simulink model "PO"  (Simulink 7.5)
settings: Solver=ode23t  StartTime=0.0  StopTime=1.4  RelTol=1e-3
libraries: powerlib x23, powerlib_extras x6, simulink x3
settings Model: Creator=Raju  LastModifiedBy=Lenovo
settings SolverCC: ZeroCrossControl=DisableAll

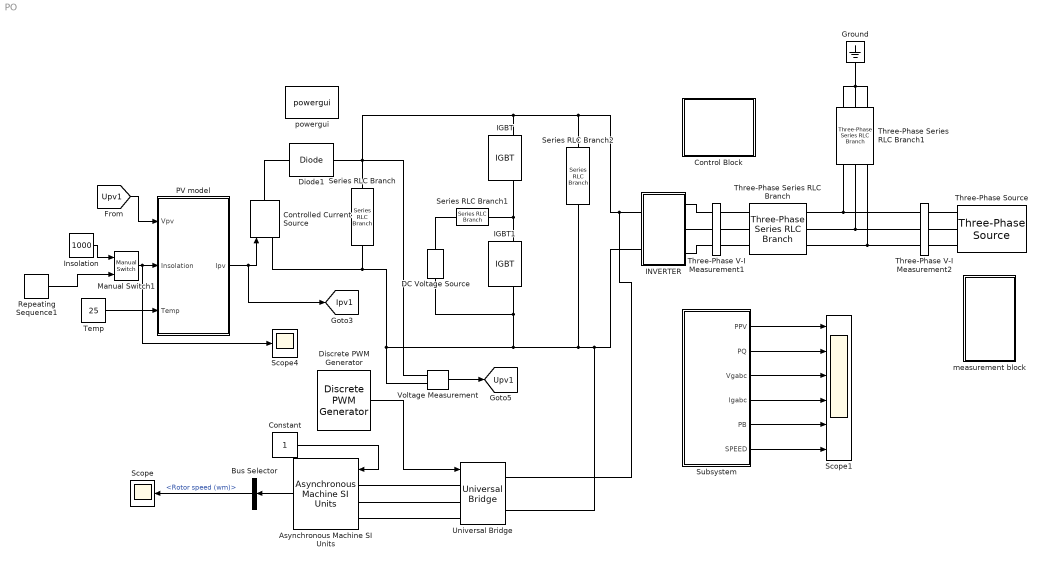
== system PO ==
  " INVERTER" : Subsystem
  Asynchronous Machine SI Units : powerlib/Machines/Asynchronous Machine SI Units  DialogController=POWERSYS.PowerSysDialog  SystemSampleTime=-1  PresetModel=No  MechanicalLoad=Torque Tm  ShowDetailedParameters=on  RotorType=Squirrel-cage  ReferenceFrame=Rotor  NominalParameters=[ 2250*746, 400, 50 ]  Stator=[ 0.029 0.226/377]  Rotor=[ 0.022 0.226/377]  Lm=13.04/377  Mechanical=[ 63.87 0 2]  PolePairs=2  InitialConditions=[1 0 0 0 0 0 0 0]  Units=SI  LoadFlowParameters=1492000  SimulateSaturation=off  Saturation=[14.03593122, 27.81365428, 53.79336849, 72.68890987, 97.98006896, 148.6815601, 215.7428561, 302.9841135, 428.7778367 ; 230, 322, 414, 460, 506, 552, 598, 644, 690]  TsPowergui=0  TsBlock=-1  IterativeModel=Forward Euler
  Bus Selector : BusSelector  OutputSignals=Mechanical.Rotor speed (wm)
  Constant : Constant  OutDataType=fixdt(1, 16)  OutScaling=2^0
  Control Block : Subsystem
  Controlled Current Source : powerlib/Electrical Sources/Controlled Current Source  DialogController=POWERSYS.PowerSysDialog  SystemSampleTime=-1  Initialize=on  Source_Type=AC  Amplitude=0  Phase=0  Frequency=0  Measurements=Current
  DC Voltage Source : powerlib/Electrical Sources/DC Voltage Source  DialogController=POWERSYS.PowerSysDialog  SystemSampleTime=-1  Amplitude=240  Measurements=None
  Diode1 : powerlib/Power Electronics/Diode  DialogController=POWERSYS.PowerSysDialog  SystemSampleTime=-1  Ron=0.001  Lon=0  Vf=0.8  IC=0  UseSnubber=off  Rs=500  Cs=250e-9  Measurements=off
  Discrete PWM Generator : powerlib_extras/Discrete  Control Blocks/Discrete PWM Generator  DialogController=POWERSYS.PowerSysDialog  SystemSampleTime=-1  GeneratorMode="3-arm  bridge (6 pulses)"  Fc=1080  Ts=50e-6  Internal=on  mIndex=0.4  Freq=60  Phase=0
  Ground : powerlib/Elements/Ground  DialogController=POWERSYS.PowerSysDialog  PhysicalDomain=powersysdomain  SubClassName=unknown  LeftPortType=p1  RightPortType=p1  LConnTagsString=a
  IGBT : powerlib/Power Electronics/IGBT  DialogController=POWERSYS.PowerSysDialog  SystemSampleTime=-1  Ron=0.001  Lon=0  Vf=1  Tf=1e-6  Tt=2e-6  IC=0  Rs=1e5  Cs=inf  Measurements=on
  IGBT1 : powerlib/Power Electronics/IGBT  DialogController=POWERSYS.PowerSysDialog  SystemSampleTime=-1  Ron=0.001  Lon=0  Vf=1  Tf=1e-6  Tt=2e-6  IC=0  Rs=1e5  Cs=inf  Measurements=on
  Insolation : Constant  Value=1000
  Manual Switch1 : simulink/Signal Routing/Manual Switch  SystemSampleTime=-1  sw=1  action=0  varsize=off
  PV model : Subsystem
  Repeating Sequence1 : simulink/Sources/Repeating Sequence  SystemSampleTime=-1  rep_seq_t=[0 0.5 0.5 0.8 0.8 1.5 ]  rep_seq_y=[1000 1000 700 700 1000 1000]
  Scope : Scope
  Scope1 : Scope  NumInputPorts=6
      settings: YMin=-5~-5~-5~-5~-5~-5  YMax=5~5~5~5~5~5  SaveName=ScopeData2
  Scope4 : Scope
      settings: YMin=-100  YMax=800  SaveName=v1
  Series RLC Branch : powerlib/Elements/Series RLC Branch  DialogController=POWERSYS.PowerSysDialog  PhysicalDomain=powersysdomain  SubClassName=unknown  LeftPortType=p1  RightPortType=p1  LConnTagsString=__new0  RConnTagsString=__new0  BranchType=C  Resistance=1  Inductance=1e-3  SetiL0=off  InitialCurrent=0  Capacitance=138e-6  Setx0=off  InitialVoltage=0  Measurements=None
  Series RLC Branch1 : powerlib/Elements/Series RLC Branch  DialogController=POWERSYS.PowerSysDialog  PhysicalDomain=powersysdomain  SubClassName=unknown  LeftPortType=p1  RightPortType=p1  LConnTagsString=__new0  RConnTagsString=__new0  BranchType=L  Resistance=1  Inductance=2.2e-3  SetiL0=off  InitialCurrent=0  Capacitance=4700e-6  Setx0=off  InitialVoltage=0  Measurements=None
  Series RLC Branch2 : powerlib/Elements/Series RLC Branch  DialogController=POWERSYS.PowerSysDialog  PhysicalDomain=powersysdomain  SubClassName=unknown  LeftPortType=p1  RightPortType=p1  LConnTagsString=__new0  RConnTagsString=__new0  BranchType=C  Resistance=1  Inductance=1e-3  SetiL0=off  InitialCurrent=0  Capacitance=4700e-6  Setx0=off  InitialVoltage=0  Measurements=None
  Subsystem : Subsystem
  Temp : Constant  Value=25
  Three-Phase Series RLC Branch : powerlib/Elements/Three-Phase Series RLC Branch  DialogController=POWERSYS.PowerSysDialog  PhysicalDomain=powersysdomain  SubClassName=unknown  LeftPortType=p1  RightPortType=p1  LConnTagsString=A|B|C  RConnTagsString=A|B|C  BranchType=L  Resistance=0.5  Inductance=6e-3  Capacitance=1e-6  Measurements=None
  Three-Phase Series RLC Branch1 : powerlib/Elements/Three-Phase Series RLC Branch  DialogController=POWERSYS.PowerSysDialog  PhysicalDomain=powersysdomain  SubClassName=unknown  LeftPortType=p1  RightPortType=p1  LConnTagsString=A|B|C  RConnTagsString=A|B|C  BranchType=RC  Resistance=1  Inductance=1e-3  Capacitance=1e-6  Measurements=None
  Three-Phase V-I Measurement1 : powerlib/Measurements/Three-Phase V-I Measurement  DialogController=POWERSYS.PowerSysDialog  SystemSampleTime=-1  VoltageMeasurement=phase-to-ground  SetLabelV=on  LabelV=Viabc  Vpu=off  VpuLL=off  CurrentMeasurement=yes  SetLabelI=on  LabelI=Iiabc  Ipu=off  Pbase=100e6  Vbase=500e3  OutputType=Complex  PhasorSimulation=off  PSBequivalent=0
      link override Model/VI/Ia: GotoTag=LibraryTag_Ia
      link override Model/VI/Ib: GotoTag=LibraryTag_Ib
      link override Model/VI/Ic: GotoTag=LibraryTag_Ic
      link override Model/VI/Va: GotoTag=LibraryTag_Va
      link override Model/VI/Vb: GotoTag=LibraryTag_Vb
      link override Model/VI/Vc: GotoTag=LibraryTag_Vc
  Three-Phase V-I Measurement2 : powerlib/Measurements/Three-Phase V-I Measurement  DialogController=POWERSYS.PowerSysDialog  SystemSampleTime=-1  VoltageMeasurement=phase-to-phase  SetLabelV=on  LabelV=Vsabc  Vpu=off  VpuLL=off  CurrentMeasurement=yes  SetLabelI=on  LabelI=Isabc  Ipu=off  Pbase=100e6  Vbase=500e3  OutputType=Complex  PhasorSimulation=off  PSBequivalent=0
      link override Model/VI/Ia: GotoTag=LibraryTag_Ia
      link override Model/VI/Ib: GotoTag=LibraryTag_Ib
      link override Model/VI/Ic: GotoTag=LibraryTag_Ic
      link override Model/VI/Va: GotoTag=LibraryTag_Va
      link override Model/VI/Vb: GotoTag=LibraryTag_Vb
      link override Model/VI/Vc: GotoTag=LibraryTag_Vc
  Three-Phase Source : powerlib/Electrical Sources/Three-Phase Source  DialogController=POWERSYS.PowerSysDialog  SystemSampleTime=-1  Voltage=400  PhaseAngle=0  Frequency=50  InternalConnection=Yg  SpecifyImpedance=off  Resistance=0.01  Inductance=2e-6  ShortCircuitLevel=10e6  BaseVoltage=400  XRratio=7
  Universal Bridge : powerlib/Power Electronics/Universal Bridge  DialogController=POWERSYS.PowerSysDialog  SystemSampleTime=-1  Arms=3  SnubberResistance=1e5  SnubberCapacitance=inf  Device=IGBT / Diodes  Ron=1e-3  Lon=0  ForwardVoltages="[  0  0  ]"  ForwardVoltage=0  GTOparameters=[ 10e-6 , 20e-6 ]  IGBTparameters=[ 1e-6 , 2e-6 ]  Measurements=None  Measurements_2=None  converterType=Rectifier
  Voltage Measurement : powerlib/Measurements/Voltage Measurement  DialogController=POWERSYS.PowerSysDialog  SystemSampleTime=-1  PhasorSimulation=off  OutputType=Complex  PSBequivalent=0
  measurement block : Subsystem
  powergui : powerlib/powergui  Priority=1  SystemSampleTime=-1  SimulationMode=Discrete  SampleTime=50e-6  frequency=60  SPID=off  DisableSnubberDevices=off  DisableRonSwitches=off  DisableVfSwitches=off  SwTol=0  Interpol=off  frequencyindice=50  echomessages=off  HookPort=off  DisplayEquations=off  FunctionMessages=off  EnableUseOfTLC=off  x0status=blocks  RestoreLinks=warning  ResistiveCurrentMeasurement=off  Ylog=off  Xlog=on  ShowGrid=off  save=off  variable=ZData  structure=Is  ZoomFFT=off  StartTime=0.5  cycles=1  DisplayStyle=1  fundamental=50  FreqAxis=on  MaxFrequency=5000  frequencyindicesteady=1  display=off  methode=off
  tag scope: Ipv1=global, Upv1=global
  wires:
  PV model/1(Ipv) -> Controlled Current Source/1, [Ipv1]
  Voltage Measurement/1 -> [Upv1]
  Temp/1 -> PV model/3(Temp)
  Manual Switch1/1 -> PV model/2(Insolation), Scope4/1
  Insolation/1 -> Manual Switch1/1
  Repeating Sequence1/1 -> Manual Switch1/2
  [Upv1] -> PV model/1(Vpv)
  Discrete PWM Generator/1 -> Universal Bridge/1
  Asynchronous Machine SI Units/1 -> Bus Selector/1
  Bus Selector/1 -> Scope/1  "<Rotor speed (wm)>"
  Constant/1 -> Asynchronous Machine SI Units/1
  Subsystem/1(PPV) -> Scope1/1
  Subsystem/2(PQ) -> Scope1/2
  Subsystem/3(Vgabc) -> Scope1/3
  Subsystem/4(Igabc) -> Scope1/4
  Subsystem/5(PB) -> Scope1/5
  Subsystem/6(SPEED) -> Scope1/6
  connections:
  Series RLC Branch2/RConn1 -- IGBT1/RConn1 -- DC Voltage Source/LConn1 -- Voltage Measurement/LConn2 -- Controlled Current Source/LConn1 -- Series RLC Branch/RConn1 -- " INVERTER"/LConn2 -- Universal Bridge/RConn2
  " INVERTER"/RConn1 -- Three-Phase V-I Measurement1/LConn1
  " INVERTER"/RConn2 -- Three-Phase V-I Measurement1/LConn2
  " INVERTER"/RConn3 -- Three-Phase V-I Measurement1/LConn3
  Three-Phase V-I Measurement1/RConn1 -- Three-Phase Series RLC Branch/LConn1
  Three-Phase V-I Measurement1/RConn2 -- Three-Phase Series RLC Branch/LConn2
  Three-Phase V-I Measurement1/RConn3 -- Three-Phase Series RLC Branch/LConn3
  Three-Phase Source/RConn1 -- Three-Phase V-I Measurement2/RConn1
  Three-Phase Source/RConn2 -- Three-Phase V-I Measurement2/RConn2
  Three-Phase Source/RConn3 -- Three-Phase V-I Measurement2/RConn3
  Three-Phase Series RLC Branch1/LConn3 -- Three-Phase Series RLC Branch/RConn3 -- Three-Phase V-I Measurement2/LConn3
  Three-Phase Series RLC Branch1/LConn2 -- Three-Phase Series RLC Branch/RConn2 -- Three-Phase V-I Measurement2/LConn2
  Three-Phase Series RLC Branch1/LConn1 -- Three-Phase Series RLC Branch/RConn1 -- Three-Phase V-I Measurement2/LConn1
  Universal Bridge/RConn1 -- Diode1/RConn1 -- Voltage Measurement/LConn1 -- Series RLC Branch/LConn1 -- IGBT/LConn1 -- Series RLC Branch2/LConn1 -- " INVERTER"/LConn1
  Diode1/LConn1 -- Controlled Current Source/RConn1
  IGBT/RConn1 -- IGBT1/LConn1 -- Series RLC Branch1/LConn1
  DC Voltage Source/RConn1 -- Series RLC Branch1/RConn1
  Universal Bridge/LConn1 -- Asynchronous Machine SI Units/LConn1
  Universal Bridge/LConn2 -- Asynchronous Machine SI Units/LConn2
  Universal Bridge/LConn3 -- Asynchronous Machine SI Units/LConn3
  Ground/LConn1 -- Three-Phase Series RLC Branch1/RConn1 -- Three-Phase Series RLC Branch1/RConn3 -- Three-Phase Series RLC Branch1/RConn2

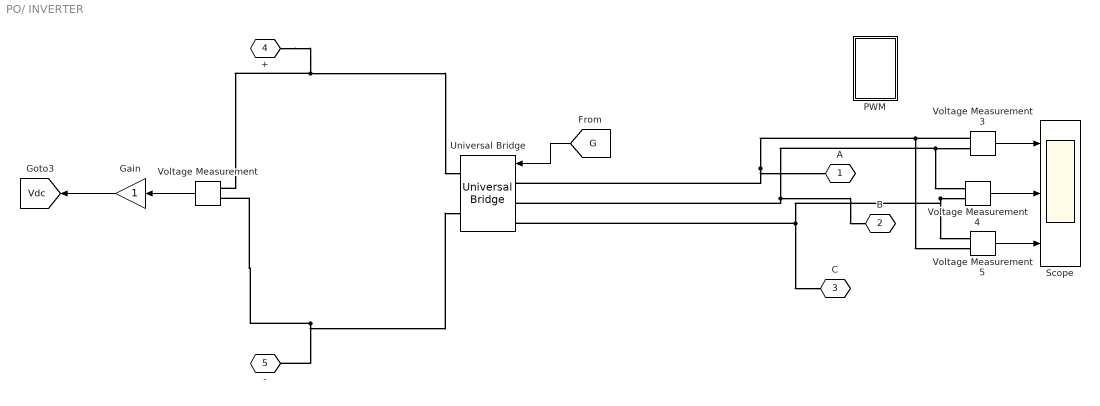
== system PO/ INVERTER ==
  Gain : Gain
  PWM : Subsystem
  Scope : Scope  NumInputPorts=3
      settings: TimeRange=0.1485544839330016  YMin=-300~-400~-300  YMax=300~300~300  SaveName=ScopeData3
  Universal Bridge : powerlib/Power Electronics/Universal Bridge  DialogController=POWERSYS.PowerSysDialog  SystemSampleTime=-1  Arms=3  SnubberResistance=1e5  SnubberCapacitance=inf  Device=IGBT / Diodes  Ron=1e-3  Lon=0  ForwardVoltages="[  0  0  ]"  ForwardVoltage=0  GTOparameters=[ 10e-6 , 20e-6 ]  IGBTparameters=[ 1e-6 , 2e-6 ]  Measurements=None  Measurements_2=None  converterType=Rectifier
  Voltage Measurement{,3..5} (4 alike) : powerlib/Measurements/Voltage Measurement  DialogController=POWERSYS.PowerSysDialog  SystemSampleTime=-1  PhasorSimulation=off  OutputType=Complex  PSBequivalent=0
  A : PMIOPort  Tag=PMCPort  Port=1  Side=Right
  B : PMIOPort  Tag=PMCPort  Port=2  Side=Right
  C : PMIOPort  Tag=PMCPort  Port=3  Side=Right
  + : PMIOPort  Tag=PMCPort  Port=4  Side=Left
  - : PMIOPort  Tag=PMCPort  Port=5  Side=Left
  tag scope: Vdc=global
  wires:
  Voltage Measurement3/1 -> Scope/1
  Voltage Measurement4/1 -> Scope/2
  Voltage Measurement5/1 -> Scope/3
  Voltage Measurement/1 -> Gain/1
  Gain/1 -> [Vdc]
  [G] -> Universal Bridge/1
  connections:
  +/RConn1 -- Voltage Measurement/LConn1 -- Universal Bridge/RConn1
  -/RConn1 -- Voltage Measurement/LConn2 -- Universal Bridge/RConn2
  Voltage Measurement4/LConn2 -- Voltage Measurement5/LConn1 -- C/RConn1 -- Universal Bridge/LConn3
  Voltage Measurement3/LConn2 -- Voltage Measurement4/LConn1 -- B/RConn1 -- Universal Bridge/LConn2
  Voltage Measurement3/LConn1 -- Voltage Measurement5/LConn2 -- A/RConn1 -- Universal Bridge/LConn1

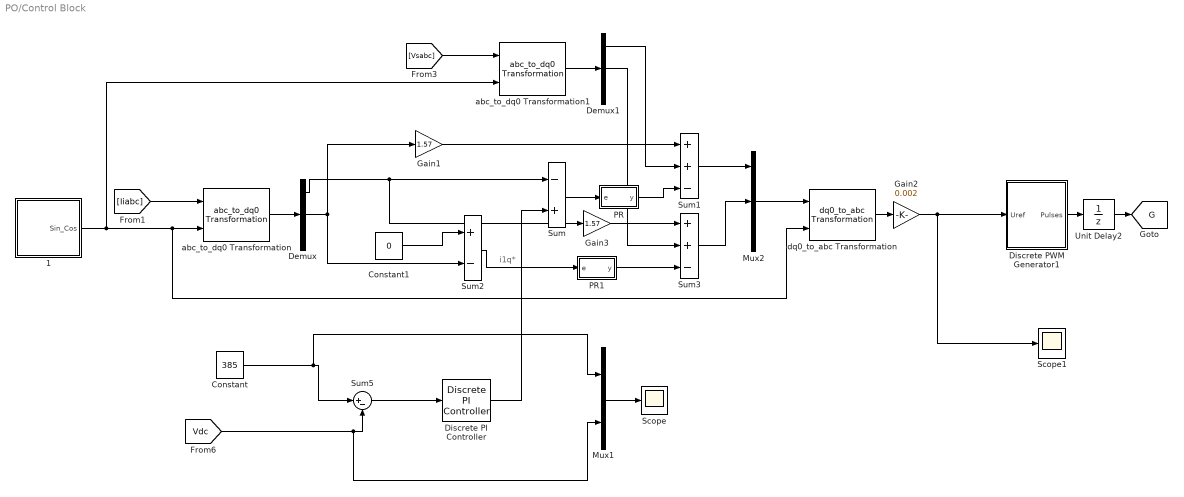
== system PO/Control Block ==
  note: i1q*
  1 : Subsystem
  Constant : Constant  Value=385  OutDataType=fixdt(1, 16)  OutScaling=2^0
  Constant1 : Constant  Value=0  OutDataType=fixdt(1, 16)  OutScaling=2^0
  Demux : Demux  Outputs=3
  Demux1 : Demux  Outputs=3
  Discrete PI Controller : powerlib_extras/Discrete  Control Blocks/Discrete PI Controller  DialogController=POWERSYS.PowerSysDialog  SystemSampleTime=-1  Kp=0.1  Ki=1  Par_Limits=[1e6 -1e6]  Init=0  Ts=50e-6
  Discrete PWM Generator1 : Subsystem  AncestorBlock=|  DialogController=POWERSYS.PowerSysDialog  mask(Discrete PWM Generator){GeneratorMode=3-arm  bridge (6 pulses), Fc=7000, Ts=50e-6, Internal=off, mIndex=0.4, Freq=60, Phase=0}
      | powerlib_extras/Discrete 
      | Control Blocks/Discrete
      | PWM Generator
      mask prompts: GeneratorMode "Generator Mode"; Fc "Carrier frequency (Hz):"; Ts "Sample time:"; Internal "Internal generation of modulating signal(s)"; mIndex "Modulation index  (0<m<1) :"; Freq "Frequency of output voltage (Hz)"; Phase "Phase of output voltage (degrees)"
      mask help:
      | This discrete block generates pulses for carrier-based PWM (Pulse Width Modulation), self-commutated IGBTs,GTOs or FETs bridges.
      |
      | Depending on the number of bridge arms selected in the "Generator Mode" parameter, the block can be used either for single-phase or three-phase PWM control.
      mask init:
      | powericon('psbcallbacks',gcb,'Discrete PWM Generator');
      | if Freq==0
      |     Phase=90;
      | end
      | switch GeneratorMode
      | case 1,
      |     Internal_Phase=0;
      |    Signal_PortWidth=1;
      |    Select1_Elements=[1 2];
      |    Select1_PortWidth=2;
      |    Select3_Elements=[1 2];
      |    Select3_PortWidth=4;
      | case 2,
      |     Internal_Phase=0;
      |     Signal_PortWidth=1;
      |     Select1_Elements=[1 2];
      |     Select1_PortWidth=2;
      |     Select3_Elements=[1 2 3 4];
      |     Select3_PortWidth=4;
      | case 3,
      |     Internal_Phase=[0 -2*pi/3 2*pi/3];
      |     Signal_PortWidth=3;
      |     Select1_Elements=[1 4 2 5 3 6];
      |     Select1_PortWidth=6;
      |    Select3_Elements=[1 2 3 4 5 6];
      |    Select3_PortWidth=12;
      | case 4,
      |     Internal_Phase=[0 -2*pi/3 2*pi/3];
      |     Signal_PortWidth=3;
      |     Select1_Elements=[1 4 2 5 3 6];
      |     Select1_PortWidth=6;
      |    Select3_Elements=[1 2 3 4 5 6 7 8 9 10 11 12];
      |    Select3_PortWidth=12;
      | end
      | power_initmask();
      mask Help:
      | The output pulses are a vector (with values=0 or 1). Depending on the selected "Generator Mode", the output vector contains:
      | For a 1-arm  bridge: Two pulses. Pulse 1 is for the upper switch and pulse 2 is for the lower switch.
      | For a 2-arm  bridge: Four pulses. Pulses 1 and 3 are respectively for the upper switches of the first and second arm. Pulses 2 and 4 are for the lower switches.
      | For a 3-arm  bridge: Six pulses. Pulses 1,3 and 5 are respectively for the upper switches of the first,second and third arm. Pulses 2,4 and 6 are for the lower switches.
      | For double 3-arm bridges: Twelve pulses.The first six pulses (pulses 1 to 6) must be sent to the first 3-arm bridge and the last six (pulses 7 to 12) to the second 3-arm bridge.
      | 
      | By selecting "Internal generation" you can can control the modulation index m, frequency and phase of the output voltage  from the internal parameters (m, Freq and Phase). Otherwise, external signals are used for pulse generation. The width of the input vector must be 1 for single phase bridges ( 1-arm or 2-arm)  and 3 for 3-phase bridges  (single or double bridge).
      mask StyleString: popup(1-arm  bridge (2 pulses)|2-arm  bridge (4 pulses)|3-arm  bridge (6 pulses)|Double 3-arm  bridges (12 pulses)),edit,edit,checkbox,edit,edit,edit
      mask CallbackString: |||%powericon('psbcallbacks',gcb,'Discrete PWM Generator',[]);|||
      mask Display: disp('')
  Gain1 : Gain  Gain=1.57
  Gain2 : Gain  Gain=0.002
  Gain3 : Gain  Gain=1.57
  Mux1 : Mux  Inputs=2
  Mux2 : Mux  Inputs=3
  PR : Subsystem
  PR1 : Subsystem
  Scope : Scope
  Scope1 : Scope
      settings: YMin=-100  YMax=800  SaveName=VPV2
  Sum : Sum  Inputs=-+
  Sum1 : Sum  Inputs=++-
  Sum2 : Sum  Inputs=+-
  Sum3 : Sum  Inputs=++-
  Sum5 : Sum  Inputs=|+-
  Unit Delay2 : UnitDelay  SampleTime=-1
  abc_to_dq0 Transformation : powerlib_extras/Measurements/abc_to_dq0 Transformation  DialogController=POWERSYS.PowerSysDialog  SystemSampleTime=-1
  abc_to_dq0 Transformation1 : powerlib_extras/Measurements/abc_to_dq0 Transformation  DialogController=POWERSYS.PowerSysDialog  SystemSampleTime=-1
  dq0_to_abc Transformation : powerlib_extras/Measurements/dq0_to_abc Transformation  DialogController=POWERSYS.PowerSysDialog  SystemSampleTime=-1
  tag scope: G=global
  wires:
  Discrete PI Controller/1 -> Sum/2
  1/1(Sin_Cos) -> abc_to_dq0 Transformation1/2, abc_to_dq0 Transformation/2, dq0_to_abc Transformation/2
  Demux/1 -> Gain3/1, Sum/1
  Constant/1 -> Sum5/1, Mux1/1
  [Iiabc] -> abc_to_dq0 Transformation/1
  abc_to_dq0 Transformation/1 -> Demux/1
  Mux2/1 -> dq0_to_abc Transformation/1
  Sum/1 -> PR/1(e)
  Sum2/1 -> PR1/1(e)
  Demux/2 -> Gain1/1, Sum2/2
  Demux1/1 -> Sum1/2
  Gain1/1 -> Sum1/1
  Demux1/2 -> Sum3/2
  Gain3/1 -> Sum3/1
  Sum1/1 -> Mux2/1
  Sum3/1 -> Mux2/2
  [Vsabc] -> abc_to_dq0 Transformation1/1
  abc_to_dq0 Transformation1/1 -> Demux1/1
  PR1/1(y) -> Sum3/3
  PR/1(y) -> Sum1/3
  [Vdc] -> Sum5/2, Mux1/2
  dq0_to_abc Transformation/1 -> Gain2/1
  Gain2/1 -> Scope1/1, Discrete PWM Generator1/1(Uref)
  Mux1/1 -> Scope/1
  Constant1/1 -> Sum2/1
  Discrete PWM Generator1/1(Pulses) -> Unit Delay2/1
  Unit Delay2/1 -> [G]
  Sum5/1 -> Discrete PI Controller/1

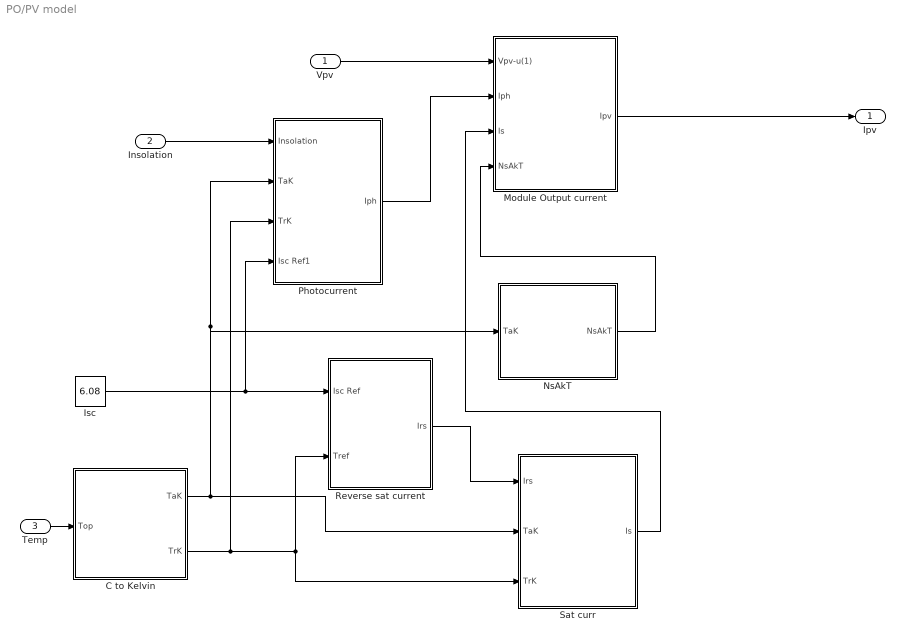
== system PO/PV model ==
  Vpv : Inport
  Insolation : Inport  Port=2
  Temp : Inport  Port=3
  C to Kelvin : Subsystem
  Isc : Constant  Value=6.08
  Module Output current : Subsystem
  NsAkT : Subsystem
  Photocurrent : Subsystem
  Reverse sat current : Subsystem
  Sat curr : Subsystem
  Ipv : Outport
  wires:
  Isc/1 -> Photocurrent/4(Isc Ref1), Reverse sat current/1(Isc Ref)
  Vpv/1 -> Module Output current/1(Vpv-u(1))
  Temp/1 -> C to Kelvin/1(Top)
  Insolation/1 -> Photocurrent/1(Insolation)
  Module Output current/1(Ipv) -> Ipv/1
  C to Kelvin/1(TaK) -> NsAkT/1(TaK), Photocurrent/2(TaK), Sat curr/2(TaK)
  Reverse sat current/1(Irs) -> Sat curr/1(Irs)
  C to Kelvin/2(TrK) -> Photocurrent/3(TrK), Sat curr/3(TrK), Reverse sat current/2(Tref)
  Sat curr/1(Is) -> Module Output current/3(Is)
  NsAkT/1(NsAkT) -> Module Output current/4(NsAkT)
  Photocurrent/1(Iph) -> Module Output current/2(Iph)

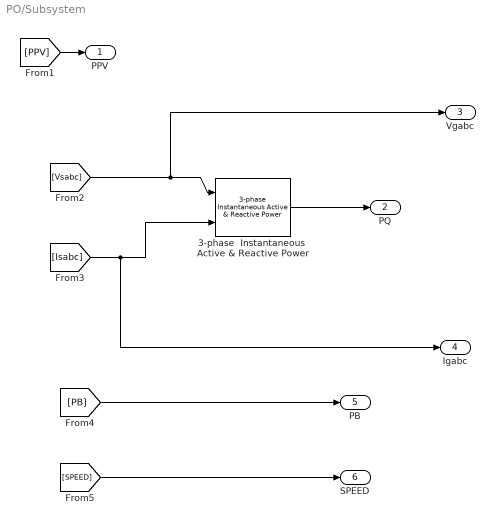
== system PO/Subsystem ==
  3-phase  Instantaneous  Active & Reactive Power : powerlib_extras/Measurements/3-phase  Instantaneous  Active & Reactive Power  DialogController=POWERSYS.PowerSysDialog  SystemSampleTime=-1
  PPV : Outport
  PQ : Outport  Port=2
  Vgabc : Outport  Port=3
  Igabc : Outport  Port=4
  PB : Outport  Port=5
  SPEED : Outport  Port=6
  wires:
  [PPV] -> PPV/1
  [Vsabc] -> 3-phase  Instantaneous  Active & Reactive Power/1, Vgabc/1
  [Isabc] -> 3-phase  Instantaneous  Active & Reactive Power/2, Igabc/1
  3-phase  Instantaneous  Active & Reactive Power/1 -> PQ/1
  [PB] -> PB/1
  [SPEED] -> SPEED/1

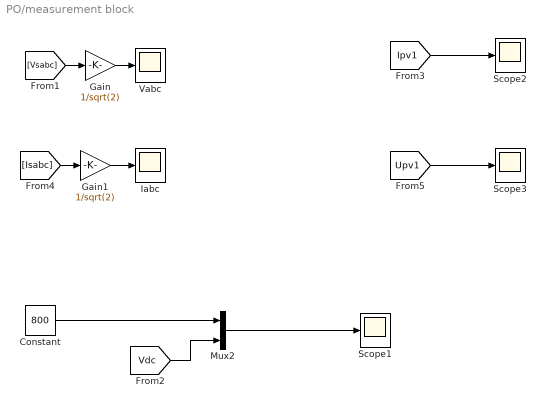
== system PO/measurement block ==
  Constant : Constant  Value=800  OutDataType=fixdt(1, 16)  OutScaling=2^0
  Gain : Gain  Gain=1/sqrt(2)  ParameterDataType=fixdt(1, 16)  ParameterScaling=2^0  OutDataType=fixdt(1, 16)  OutScaling=2^0
  Gain1 : Gain  Gain=1/sqrt(2)  ParameterDataType=fixdt(1, 16)  ParameterScaling=2^0  OutDataType=fixdt(1, 16)  OutScaling=2^0
  Iabc : Scope
      settings: YMin=-500  YMax=500  SaveName=Is
  Mux2 : Mux  Inputs=2
  Scope1 : Scope
      settings: TimeRange=1.4  YMin=0  YMax=900  SaveName=Vdc
  Scope2 : Scope
      settings: TimeRange=1.4  YMin=-100  YMax=100  SaveName=Vdc1
  Scope3 : Scope
      settings: TimeRange=1.4  YMin=-100  YMax=100  SaveName=Vdc2
  Vabc : Scope
      settings: TimeRange=1  YMin=-600  YMax=600  SaveName=Vs
  wires:
  [Vsabc] -> Gain/1
  [Isabc] -> Gain1/1
  Mux2/1 -> Scope1/1
  Constant/1 -> Mux2/1
  [Vdc] -> Mux2/2
  Gain/1 -> Vabc/1
  Gain1/1 -> Iabc/1
  [Ipv1] -> Scope2/1
  [Upv1] -> Scope3/1

== system PO/ INVERTER/PWM ==

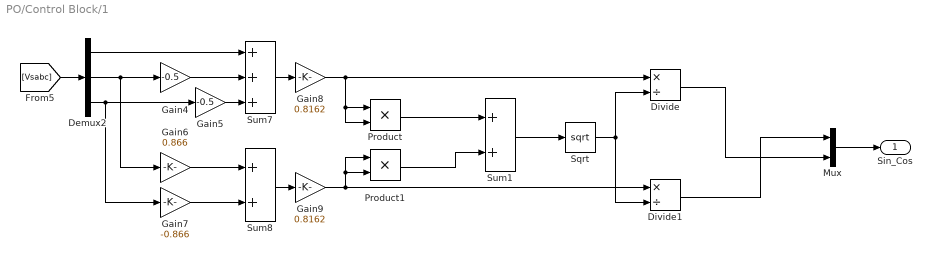
== system PO/Control Block/1 ==
  Demux2 : Demux  Outputs=3
  Divide : Product  Inputs=*/
  Divide1 : Product  Inputs=*/
  Gain4 : Gain  Gain=-0.5
  Gain5 : Gain  Gain=-0.5
  Gain6 : Gain  Gain=0.866
  Gain7 : Gain  Gain=-0.866
  Gain8 : Gain  Gain=0.8162
  Gain9 : Gain  Gain=0.8162
  Mux : Mux  Inputs=2
  Product : Product  RndMeth=Zero
  Product1 : Product  RndMeth=Zero
  Sqrt : Sqrt  SaturateOnIntegerOverflow=on
  Sum1 : Sum
  Sum7 : Sum  Inputs=+++
  Sum8 : Sum
  Sin_Cos : Outport
  wires:
  Demux2/1 -> Sum7/1
  Demux2/2 -> Gain4/1, Gain6/1
  Demux2/3 -> Gain5/1, Gain7/1
  Gain4/1 -> Sum7/2
  Gain5/1 -> Sum7/3
  Sum7/1 -> Gain8/1
  Gain6/1 -> Sum8/1
  Gain7/1 -> Sum8/2
  Sum8/1 -> Gain9/1
  Gain8/1 -> Product/1, Product/2, Divide/1
  Gain9/1 -> Product1/1, Product1/2, Divide1/1
  [Vsabc] -> Demux2/1
  Product/1 -> Sum1/1
  Product1/1 -> Sum1/2
  Sum1/1 -> Sqrt/1
  Sqrt/1 -> Divide/2, Divide1/2
  Divide1/1 -> Mux/1
  Divide/1 -> Mux/2
  Mux/1 -> Sin_Cos/1

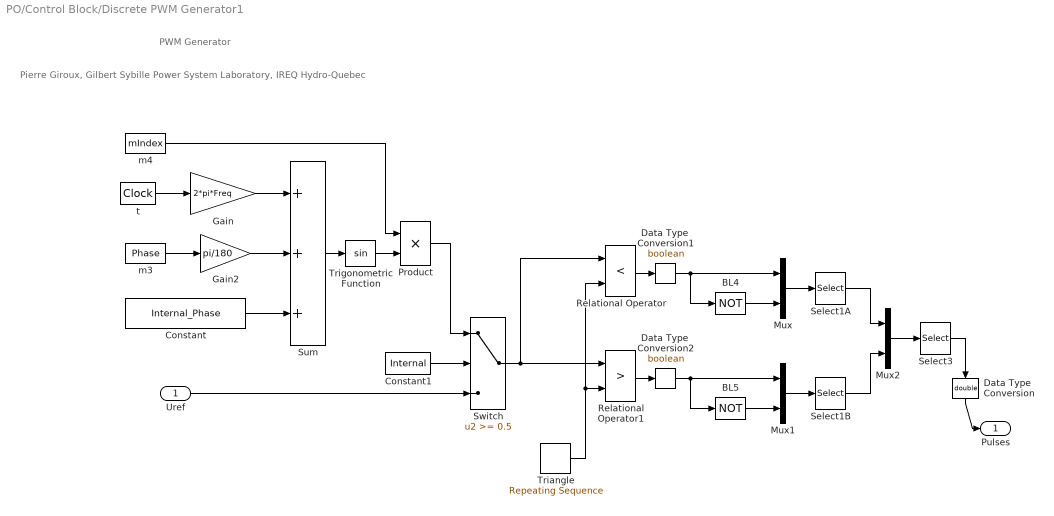
== system PO/Control Block/Discrete PWM Generator1 ==
  note: PWM Generator
  note: Pierre Giroux, Gilbert Sybille
      | Power System Laboratory, IREQ
      | Hydro-Quebec
  Uref : Inport  SampleTime=Ts  OutDataType=sfix(16)  OutScaling=2^0
  BL4 : Logic  Operator=NOT  Inputs=1  SampleTime=Ts
  BL5 : Logic  Operator=NOT  Inputs=1  SampleTime=Ts
  Constant : Constant  Value=Internal_Phase  OutDataType=sfix(16)  OutScaling=2^0  SampleTime=Ts
  Constant1 : Constant  Value=Internal  OutDataType=sfix(16)  OutScaling=2^0  SampleTime=Ts
  Data Type  Conversion : DataTypeConversion  OutDataTypeMode=double  OutDataType=sfix(16)  OutScaling=2^0  OutDataTypeStr=double  SampleTime=Ts  SaturateOnIntegerOverflow=on  RndMeth=Zero
  Data Type  Conversion1 : DataTypeConversion  OutDataTypeMode=boolean  OutDataType=sfix(16)  OutScaling=2^0  OutDataTypeStr=boolean  SampleTime=Ts  SaturateOnIntegerOverflow=on  RndMeth=Zero
  Data Type  Conversion2 : DataTypeConversion  OutDataTypeMode=boolean  OutDataType=sfix(16)  OutScaling=2^0  OutDataTypeStr=boolean  SampleTime=Ts  SaturateOnIntegerOverflow=on  RndMeth=Zero
  Gain : Gain  Gain=2*pi*Freq  ParameterDataType=sfix(16)  ParameterScaling=2^0  OutDataType=sfix(16)  OutScaling=2^0  SaturateOnIntegerOverflow=on  OutDataTypeStr=Inherit: Same as input  ParamDataTypeStr=Inherit: Same as input
  Gain2 : Gain  Gain=pi/180  ParameterDataType=sfix(16)  ParameterScaling=2^0  OutDataType=sfix(16)  OutScaling=2^0  SaturateOnIntegerOverflow=on  OutDataTypeStr=Inherit: Same as input  ParamDataTypeStr=Inherit: Same as input
  Mux : Mux  Inputs=2
  Mux1 : Mux  Inputs=2
  Mux2 : Mux  Inputs=2
  Product : Product  OutDataType=sfix(16)  OutScaling=2^0  SampleTime=Ts  SaturateOnIntegerOverflow=on  InputSameDT=on  OutDataTypeStr=Inherit: Same as first input
  Relational Operator : RelationalOperator  Operator=<  SampleTime=Ts  InputSameDT=on
  Relational Operator1 : RelationalOperator  Operator=>  SampleTime=Ts  InputSameDT=on
  Select1A : Selector  InputPortWidth=Select1_PortWidth  IndexOptions=Index vector (dialog)  Indices=Select1_Elements  OutputSizes=1
  Select1B : Selector  InputPortWidth=Select1_PortWidth  IndexOptions=Index vector (dialog)  Indices=Select1_Elements  OutputSizes=1
  Select3 : Selector  InputPortWidth=Select3_PortWidth  IndexOptions=Index vector (dialog)  Indices=Select3_Elements  OutputSizes=1
  Sum : Sum  Inputs=+++  OutDataType=sfix(16)  OutScaling=2^0  SampleTime=Ts  SaturateOnIntegerOverflow=on  InputSameDT=on  OutDataTypeStr=Inherit: Same as first input
  Switch : Switch  Threshold=0.5  OutDataType=sfix(16)  OutScaling=2^0  SampleTime=Ts  SaturateOnIntegerOverflow=on  InputSameDT=on
  Triangle : simulink/Sources/Repeating Sequence  SystemSampleTime=-1  rep_seq_t=[0 1/Fc/2 1/Fc]  rep_seq_y=[-1 1 -1]
  Trigonometric Function : Trigonometry  SampleTime=Ts
  m3 : Constant  Value=Phase  OutDataType=sfix(16)  OutScaling=2^0  SampleTime=Ts
  m4 : Constant  Value=mIndex  OutDataType=sfix(16)  OutScaling=2^0  SampleTime=Ts
  t : DigitalClock  SampleTime=Ts
  Pulses : Outport  SampleTime=Ts  OutDataType=sfix(16)  OutScaling=2^0
  wires:
  Data Type  Conversion2/1 -> Mux1/1, BL5/1
  Relational Operator1/1 -> Data Type  Conversion2/1
  Data Type  Conversion1/1 -> Mux/1, BL4/1
  Relational Operator/1 -> Data Type  Conversion1/1
  Data Type  Conversion/1 -> Pulses/1
  Select3/1 -> Data Type  Conversion/1
  t/1 -> Gain/1
  Gain/1 -> Sum/1
  Gain2/1 -> Sum/2
  m3/1 -> Gain2/1
  Constant/1 -> Sum/3
  m4/1 -> Product/1
  Sum/1 -> Trigonometric Function/1
  Trigonometric Function/1 -> Product/2
  Uref/1 -> Switch/3
  Constant1/1 -> Switch/2
  Product/1 -> Switch/1
  Triangle/1 -> Relational Operator/2, Relational Operator1/2
  BL4/1 -> Mux/2
  BL5/1 -> Mux1/2
  Mux/1 -> Select1A/1
  Mux1/1 -> Select1B/1
  Select1A/1 -> Mux2/1
  Select1B/1 -> Mux2/2
  Mux2/1 -> Select3/1
  Switch/1 -> Relational Operator/1, Relational Operator1/1

== system PO/Control Block/PR ==
  e : Inport
  Integrator : Integrator
  Ki/w : Gain  Gain=0.09/314
  Kp : Gain  Gain=0.25
  Sum4 : Sum  Inputs=|++  OutDataType=fixdt(1, 16)  OutScaling=2^0
  Sum6 : Sum  Inputs=|++  OutDataType=fixdt(1, 16)  OutScaling=2^0
  w : Gain  Gain=314
  w1 : Gain  Gain=-314
  y : Outport
  wires:
  e/1 -> Kp/1, Ki/w/1
  Ki/w/1 -> Sum4/1
  Sum4/1 -> w/1
  w/1 -> Integrator/1
  Kp/1 -> Sum6/1
  Integrator/1 -> Sum6/2, w1/1
  w1/1 -> Sum4/2
  Sum6/1 -> y/1

== system PO/Control Block/PR1 ==
  e : Inport
  Integrator : Integrator
  Ki/w : Gain  Gain=0.09/314
  Kp : Gain  Gain=0.25
  Sum4 : Sum  Inputs=|++  OutDataType=fixdt(1, 16)  OutScaling=2^0
  Sum6 : Sum  Inputs=|++  OutDataType=fixdt(1, 16)  OutScaling=2^0
  w : Gain  Gain=314
  w1 : Gain  Gain=-314
  y : Outport
  wires:
  Sum6/1 -> y/1
  w1/1 -> Sum4/2
  Integrator/1 -> w1/1, Sum6/2
  Kp/1 -> Sum6/1
  w/1 -> Integrator/1
  Sum4/1 -> w/1
  Ki/w/1 -> Sum4/1
  e/1 -> Ki/w/1, Kp/1

== system PO/PV model/C to Kelvin ==
  Top : Inport
  Sum : Sum  Inputs=|++
  Sum1 : Sum  Inputs=|++
  Tk : Constant  Value=273
  Tref : Constant  Value=25
  TaK : Outport
  TrK : Outport  Port=2
  wires:
  Sum1/1 -> TrK/1
  Sum/1 -> TaK/1
  Tref/1 -> Sum1/2
  Tk/1 -> Sum/2, Sum1/1
  Top/1 -> Sum/1

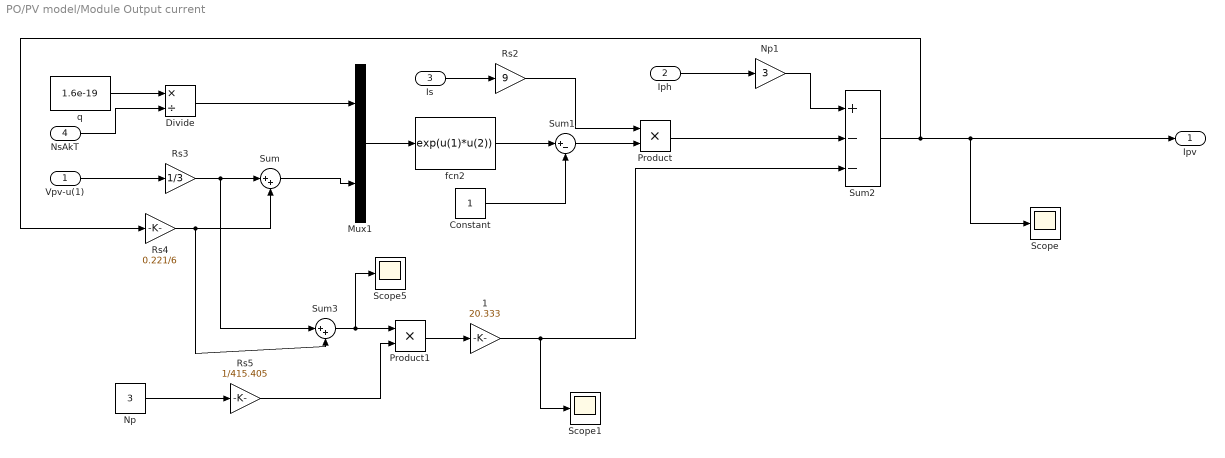
== system PO/PV model/Module Output current ==
  Vpv-u(1) : Inport
  Iph : Inport  Port=2
  Is : Inport  Port=3
  NsAkT : Inport  Port=4
  1 : Gain  Gain=20.333
  Constant : Constant  OutDataType=fixdt(1, 16)  OutScaling=2^0
  Divide : Product  Inputs=*/  OutDataType=fixdt(1, 16)  OutScaling=2^-10
  Mux1 : Mux  Inputs=2
  Np : Constant  Value=3  OutDataType=fixdt(1, 16)  OutScaling=2^0
  Np1 : Gain  Gain=3
  Product : Product  OutDataType=fixdt(1, 16)  OutScaling=2^0  RndMeth=Zero
  Product1 : Product  OutDataType=fixdt(1, 16)  OutScaling=2^0  RndMeth=Zero
  Rs2 : Gain  Gain=9
  Rs3 : Gain  Gain=1/3
  Rs4 : Gain  Gain=0.221/6
  Rs5 : Gain  Gain=1/415.405
  Scope : Scope
      settings: SaveName=ScopeData29
  Scope1 : Scope
      settings: SaveName=ScopeData30
  Scope5 : Scope
      settings: SaveName=ScopeData22
  Sum : Sum  Inputs=|++  OutDataType=fixdt(1, 16)  OutScaling=2^0
  Sum1 : Sum  Inputs=|+-  OutDataType=fixdt(1, 16)  OutScaling=2^0
  Sum2 : Sum  Inputs=+--  OutDataType=fixdt(1, 16)  OutScaling=2^0
  Sum3 : Sum  Inputs=|++  OutDataType=fixdt(1, 16)  OutScaling=2^0
  fcn2 : Fcn  Expr=exp(u(1)*u(2))
  q : Constant  Value=1.6e-19
  Ipv : Outport
  wires:
  Sum2/1 -> Rs4/1, Ipv/1, Scope/1
  Product1/1 -> 1/1
  Rs5/1 -> Product1/2
  Sum3/1 -> Product1/1, Scope5/1
  Np/1 -> Rs5/1
  Product/1 -> Sum2/2
  Rs2/1 -> Product/1
  Sum1/1 -> Product/2
  Constant/1 -> Sum1/2
  fcn2/1 -> Sum1/1
  Mux1/1 -> fcn2/1
  Sum/1 -> Mux1/2
  Rs4/1 -> Sum3/2, Sum/2
  Rs3/1 -> Sum3/1, Sum/1
  Vpv-u(1)/1 -> Rs3/1
  Divide/1 -> Mux1/1
  NsAkT/1 -> Divide/2
  q/1 -> Divide/1
  Is/1 -> Rs2/1
  Np1/1 -> Sum2/1
  Iph/1 -> Np1/1
  1/1 -> Sum2/3, Scope1/1

== system PO/PV model/NsAkT ==
  TaK : Inport
  A : Constant
  Product : Product  Inputs=4  RndMeth=Zero
  c : Constant  Value=27
  k : Constant  Value=1.38e-23
  NsAkT : Outport
  wires:
  Product/1 -> NsAkT/1
  TaK/1 -> Product/1
  c/1 -> Product/4
  A/1 -> Product/3
  k/1 -> Product/2

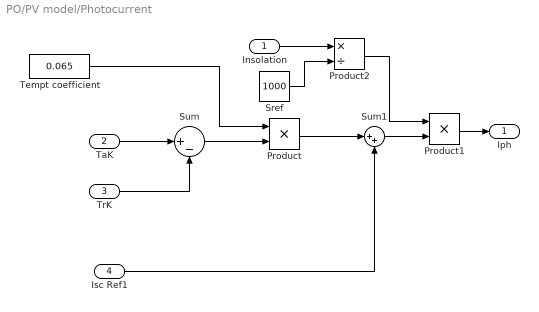
== system PO/PV model/Photocurrent ==
  Insolation : Inport
  TaK : Inport  Port=2
  TrK : Inport  Port=3
  Isc Ref1 : Inport  Port=4
  Product : Product  RndMeth=Zero
  Product1 : Product  RndMeth=Zero
  Product2 : Product  Inputs=*/  RndMeth=Zero
  Sref : Constant  Value=1000
  Sum : Sum  Inputs=|+-
  Sum1 : Sum  Inputs=|++
  Tempt coefficient : Constant  Value=0.065
  Iph : Outport
  wires:
  Product2/1 -> Product1/1
  Sref/1 -> Product2/2
  Insolation/1 -> Product2/1
  TrK/1 -> Sum/2
  TaK/1 -> Sum/1
  Product1/1 -> Iph/1
  Isc Ref1/1 -> Sum1/2
  Sum1/1 -> Product1/2
  Product/1 -> Sum1/1
  Tempt coefficient/1 -> Product/1
  Sum/1 -> Product/2

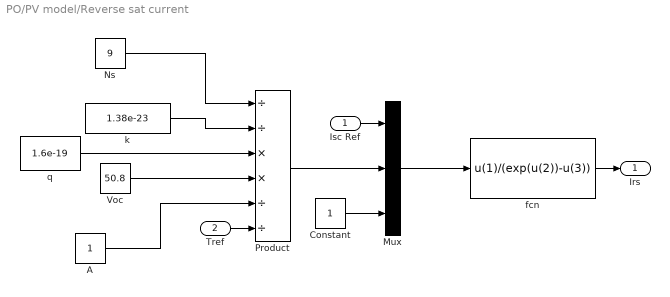
== system PO/PV model/Reverse sat current ==
  Isc Ref : Inport
  Tref : Inport  Port=2
  A : Constant
  Constant : Constant
  Mux : Mux  Inputs=3
  Ns : Constant  Value=9
  Product : Product  Inputs=//**//  RndMeth=Zero
  Voc : Constant  Value=50.8
  fcn : Fcn  Expr=u(1)/(exp(u(2))-u(3))
  k : Constant  Value=1.38e-23
  q : Constant  Value=1.6e-19
  Irs : Outport
  wires:
  Tref/1 -> Product/6
  fcn/1 -> Irs/1
  Isc Ref/1 -> Mux/1
  Mux/1 -> fcn/1
  Constant/1 -> Mux/3
  Product/1 -> Mux/2
  A/1 -> Product/5
  Voc/1 -> Product/4
  Ns/1 -> Product/1
  k/1 -> Product/2
  q/1 -> Product/3

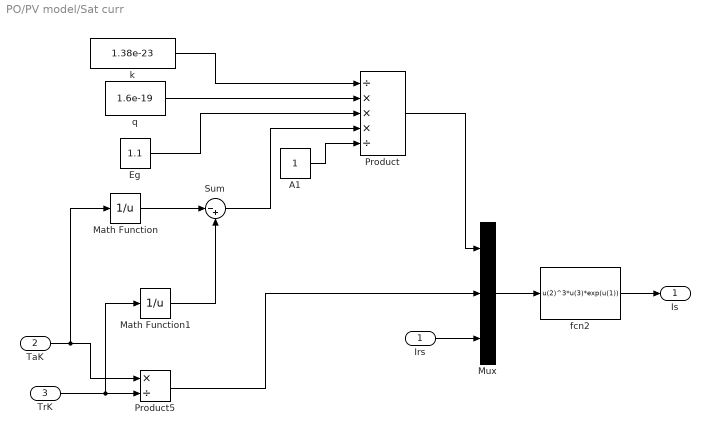
== system PO/PV model/Sat curr ==
  Irs : Inport
  TaK : Inport  Port=2
  TrK : Inport  Port=3
  A1 : Constant
  Eg : Constant  Value=1.1
  Math Function : Math  Operator=reciprocal  OutDataType=fixdt(1, 16)  OutScaling=2^0  SaturateOnIntegerOverflow=on
  Math Function1 : Math  Operator=reciprocal  OutDataType=fixdt(1, 16)  OutScaling=2^0  SaturateOnIntegerOverflow=on
  Mux : Mux  Inputs=3
  Product : Product  Inputs=/***/  RndMeth=Zero
  Product5 : Product  Inputs=*/  RndMeth=Zero
  Sum : Sum  Inputs=|-+
  fcn2 : Fcn  Expr=u(2)^3*u(3)*exp(u(1))
  k : Constant  Value=1.38e-23
  q : Constant  Value=1.6e-19
  Is : Outport
  wires:
  Math Function1/1 -> Sum/2
  Math Function/1 -> Sum/1
  Irs/1 -> Mux/3
  fcn2/1 -> Is/1
  Product5/1 -> Mux/2
  Product/1 -> Mux/1
  Mux/1 -> fcn2/1
  TaK/1 -> Math Function/1, Product5/1
  TrK/1 -> Math Function1/1, Product5/2
  A1/1 -> Product/5
  Sum/1 -> Product/4
  Eg/1 -> Product/3
  q/1 -> Product/2
  k/1 -> Product/1
